simulink model "PositionTransitionHandler"  (R2016b)
settings: Solver=FixedStepAuto  StartTime=0.0  StopTime=10.0  RelTol=1e-3  EnableMultiTasking=on
settings Model: Creator=march  LastModifiedBy=snyke7
settings SolverCC: EnableConcurrentExecution=on
settings DataIOCC: SaveFormat=StructureWithTime
settings OptimizationCC: BlockReduction=off  OptimizeBlockIOStorage=off  BufferReuse=off  GlobalBufferReuse=off  ExpressionFolding=off  LocalBlockOutputs=off
settings HardwareCC: ProdBitPerPointer=32  ProdBitPerSizeT=32  ProdBitPerPtrDiffT=32  ProdLargestAtomicFloat=None  ProdWordSize=32  ProdLongLongMode=on  ProdHWDeviceType=Generic->32-bit x86 compatible
settings RTWCC: SystemTargetFile=slrt.tlc  TemplateMakefile=slrt_default_tmf  Description=Simulink Real-Time  RTWCompilerOptimization=on
settings TargetCC: CodeReplacementLibrary=XPC_BLAS  ParMdlRefBuildCompliant=on  ConcurrentExecutionCompliant=on  GeneratePreprocessorConditionals=Use local settings  MatFileLogging=on  MATLABClassNameForMDSCustomization=xpcAperiodicCustomization

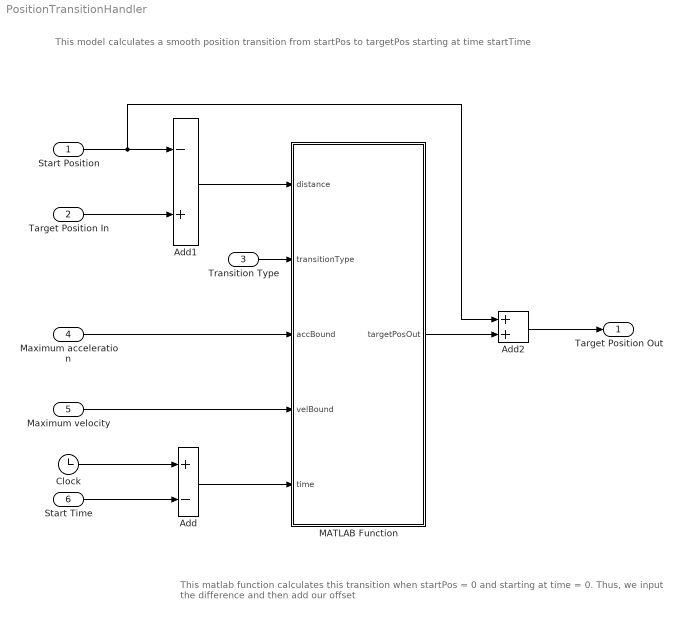
== system PositionTransitionHandler ==
  note: This matlab function calculates this transition when startPos = 0 and starting at time = 0. Thus, we input the difference and then add our offset
  note: This model calculates a smooth position transition from startPos to targetPos starting at time startTime
  Start Position : Inport
  Target Position In : Inport  Port=2
  Transition Type : Inport  Port=3
  Maximum acceleration : Inport  Port=4
  Maximum velocity : Inport  Port=5
  Start Time : Inport  Port=6
  Add : Sum  Inputs=+-
  Add1 : Sum  Inputs=-+
  Add2 : Sum
  Clock : Clock
  MATLAB Function : MATLAB Function  TreatAsAtomicUnit=on
  Target Position Out : Outport
  wires:
  Clock/1 -> Add/1
  Start Time/1 -> Add/2
  Target Position In/1 -> Add1/2
  Start Position/1 -> Add2/1, Add1/1
  Add1/1 -> MATLAB Function/1(distance)
  Transition Type/1 -> MATLAB Function/2(transitionType)
  Maximum acceleration/1 -> MATLAB Function/3(accBound)
  Maximum velocity/1 -> MATLAB Function/4(velBound)
  Add/1 -> MATLAB Function/5(time)
  MATLAB Function/1(targetPosOut) -> Add2/2
  Add2/1 -> Target Position Out/1

== matlab function PositionTransitionHandler/MATLAB Function ==
  data: distance input; targetPosOut output; transitionType input; accBound input; velBound input; time input
function targetPosOut = getTargetPosOut(distance, transitionType, accBound, velBound, time)
%% Calculates the value of a smooth transition from zero to distance at time
% Calculates the position value at time time of a smooth transition with
% maximum acceleration accBound and maximum velocity velBound
% A smooth transition is defined as arrival at the destination point with
% first derivative zero

% First, we see how long it would take to reach distance if we first
% accelerate as fast as possible and then decelerate as fast as possible
% This corresponds to p(t) = 0.5*a*t^2 untill we're halfway. Symmetry now
% takes care of reaching the destination with the desired properties. So we
% solve: 0.5*distance = 0.5*a*t^2
%       distance = a*t^2
%       t = sqrt(distance/a).
% This is the time to reach halfway so the total time needed is twice this.
% We also take the absolute value of the distance, as for negative distance
% we will use negative acceleration
timeNeeded = 2*sqrt(abs(distance)/accBound);

% To see if we can use the approach above, we check if the maximum velocity
% in this approach is higher than the velocity bound. We have
% v(t) = a*t for t <= timeNeeded/2 so the maximum velocity reached is:
maxVel = accBound*timeNeeded/2;

% note that we will correct for the sign of distance at the end of the
% function
if maxVel >= velBound 
    % In this case we have to speed up to the maximum allowed velocity,
    % then continue at a constant velocity untill we reach the point where
    % speeding down at the maximum deceleration stops us exactly at the
    % desired destination
    
    % We first calculate how long we can accelerate until we reach maximum
    % velocity. Since v(t) = at:
    timeToStopAcc = velBound/accBound;
    % The distance travelled in this time is equal to p(t) = 0.5*a*t^2
    distanceAcc = 0.5*accBound*timeToStopAcc^2;
    % Due to symmetry:
    distanceDec = distanceAcc;
    % Remaining distance to be travelled at constant velocity:
    distanceRem = abs(distance) - distanceAcc - distanceDec;
    % We now calculate the time we are at constant velocity with p(t) = vt
    timeConstantVel = distanceRem/velBound;
    % After acceleration and time at constantVel, we start decelerating:
    timeToStartDec = timeToStopAcc + timeConstantVel;
    % Finally, due to symmetry since deceleration takes the same amount of
    % time as acceleration:
    timeNeeded = timeToStartDec + timeToStopAcc;
    
    % Now we use the current time to calculate the targetPosOut.
    if time < timeToStopAcc
        % Now p(t) = 0.5 * a * t^2
        targetPosOut = 0.5 * accBound * time^2;
    elseif time < timeToStartDec
        % Then we have travelled distanceAcc, and the distance travelled at
        % constant velocity is given by p(t) = v(time - timeToStopAcc)
        travelledPos = distanceAcc;
        targetPosOut = travelledPos + velBound * (time - timeToStopAcc);
    else
        % Now we start decelerating. The travelled distance is given by
        % distanceAcc + distanceRem
        travelledPos = distanceAcc + distanceRem;
        % The velocity at a given time is equal to the maxvelocity minus
        % the acceleration times the time passed since timeToStartDec. The
        % position travelled since timeToStartDec is the integral from
        % timeToStartDec to time over this velocity. As we know the total
        % area is timeToStartAcc, we can calculate the desired area by
        % substracting the other part. That part is easy to calculate,
        % since it is the same distance as travelled when speeding up from
        % 0 to timeNeeded - time. So:
        targetPosOut = travelledPos + distanceDec - 0.5*accBound*(timeNeeded - time)^2;
    end
else
    % This means we can keep accelerating until halfway, then decelerate
    midTime = timeNeeded/2;
    if time < midTime
        % in the acceleration phase: p(t) = 0.5*a*t^2
        targetPosOut = 0.5 * accBound * time^2;
    else
        % Due to how we chose timeNeeded, we have travelled exactly half of
        % the distance
        travelledPos = abs(distance)/2;
        % Same reasoning as for the deceleration phase of the three-phase
        % way, but now distanceDec = abs(distance)/2 so that we have:
        targetPosOut = travelledPos + abs(distance)/2 - 0.5 * accBound*(timeNeeded - time)^2;
    end
end
if sign(distance) == -1
    % then negate the targetPosition, as all calculations have been done
    % with abs(distance)
    targetPosOut = -targetPosOut;
end

% finally, if time > timeNeeded (which has now correctly been set), then we
% have reached the target position
if time > timeNeeded
    targetPosOut = distance;
end
end
